simulink model "example_9_3"  (R2023b)
settings: Solver=FixedStepAuto  StartTime=0.0  StopTime=11  FixedStep=0.01  RelTol=1e-3
libraries: dspfdesign x1, simulink x1
settings Model: Creator=wangh  LastModifiedBy=wangh

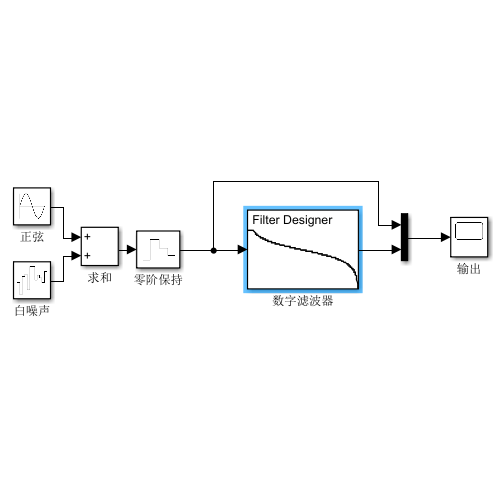
[thumbnail: Simulink's stored preview of the top-level diagram]
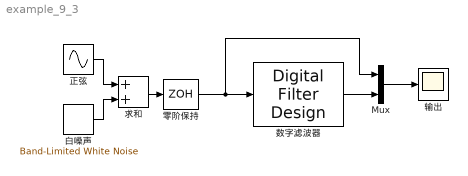
== system example_9_3 ==
  Mux : Mux  Inputs=2
  数字滤波器 : dspfdesign/Digital Filter Design  mwdsp_browser_bugfix_var=off
  正弦 : Sin  Frequency=pi  SampleTime=0
  求和 : Sum
  白噪声 : simulink/Sources/Band-Limited White Noise  Cov=[0.002]  Ts=0.01  seed=[23341]
  输出 : Scope
  零阶保持 : ZeroOrderHold  SampleTime=0.01
  wires:
  零阶保持/1 -> Mux/1, 数字滤波器/1
  正弦/1 -> 求和/1
  白噪声/1 -> 求和/2
  Mux/1 -> 输出/1
  数字滤波器/1 -> Mux/2
  求和/1 -> 零阶保持/1
